simulink model "MagnetoShield_LQ_SIMO_DUE"  (R2019a)
settings: Solver=FixedStepAuto  StartTime=0.0  StopTime=15  RelTol=1e-3  EnableMultiTasking=on
values from neighbouring files (symbols this model uses):
  A = modeld.a    [MagnetoShield_LQ_SIMO_Initialization.m]
  B = modeld.b    [MagnetoShield_LQ_SIMO_Initialization.m]
  C = modeld.c    [MagnetoShield_LQ_SIMO_Initialization.m]
  Ck = [1 0 0;0 0 1]    [MagnetoShield_LQ_SIMO_Initialization.m]
  Dk = [0;0]    [MagnetoShield_LQ_SIMO_Initialization.m]
  K = dlqr(Ai,Bi,Qlq,Rlq)    [MagnetoShield_LQ_SIMO_Initialization.m]
  R = diag([1.5815e-10,6.6217e-09])    [MagnetoShield_LQ_SIMO_Initialization.m]
  Ts = 0.0015    [MagnetoShield_LQ_SIMO_Initialization.m]
undefined symbols (not defined in the file or in its folder): DiscIntNeverNeededParam, Discrete, i0, sigbuilder_block, Time, u0, y0
libraries: MagnetoLibrary x3, ctrlSharedLib x1
settings Model: SimulationMode=external  ExtModeTrigDuration=2  Creator=Jakub  LastModifiedBy=jakub
settings OptimizationCC: EnhancedBackFolding=on  PassReuseOutputArgsAs=Individual arguments  MaxStackSize=64  OptimizeBlockOrder=speed  DifferentSizesBufferReuse=on  OptimizationCustomize=off
settings DebuggingCC: ParameterTunabilityLossMsg=error
settings HardwareCC: ProdBitPerPointer=32  ProdBitPerSizeT=32  ProdBitPerPtrDiffT=32  ProdLargestAtomicInteger=Long  ProdLargestAtomicFloat=Double  ProdWordSize=32  ProdHWDeviceType=ARM Compatible->ARM Cortex
settings SFSimCC: MATLABDynamicMemAlloc=off
settings RTWCC: SystemTargetFile=ert.tlc  HardwareBoard=Arduino Due  TLCOptions=-aInlineSetEventsForThisBaseRateFcn=TLC_FALSE -aSuppressMultiTaskScheduler=TLC_FALSE -aRateBasedStepFcn=1  TemplateMakefile=ert_default_tmf  GenerateReport=on  Toolchain=Arduino ARM  BuildConfiguration=Faster Runs  IncludeHyperlinkInReport=on  LaunchReport=on  GenerateTraceInfo=on  GenerateTraceReport=on  GenerateTraceReportSl=on  GenerateTraceReportSf=on  GenerateTraceReportEml=on
settings CodeAppCC: ForceParamTrailComments=on  IgnoreCustomStorageClasses=off  OperatorAnnotations=on  SimulinkDataObjDesc=on  SFDataObjDesc=on  InsertBlockDesc=on
settings ERTTargetCC: SupportContinuousTime=on  SupportVariableSizeSignals=on  ExtModeStaticAllocSize=24576

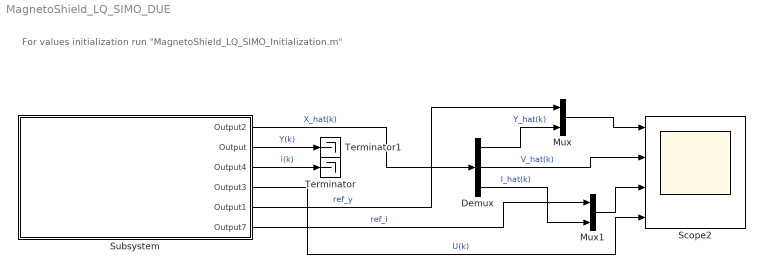
== system MagnetoShield_LQ_SIMO_DUE ==
  note: For values initialization run "MagnetoShield_LQ_SIMO_Initialization.m"
  Demux : Demux  Outputs=3
  Mux : Mux  Inputs=2
  Mux1 : Mux  Inputs=2
  Scope2 : Scope  NumInputPorts=4
  Subsystem : Subsystem
  Terminator : Terminator
  Terminator1 : Terminator
  wires:
  Subsystem/2(Output) -> Terminator1/1  "Y(k)"
  Demux/2 -> Scope2/2  "V_hat(k)"
  Demux/3 -> Mux1/2  "I_hat(k)"
  Mux1/1 -> Scope2/3
  Mux/1 -> Scope2/1
  Demux/1 -> Mux/2  "Y_hat(k)"
  Subsystem/1(Output2) -> Demux/1  "X_hat(k)"
  Subsystem/4(Output3) -> Scope2/4  "U(k)"
  Subsystem/6(Output7) -> Mux1/1  "ref_i"
  Subsystem/5(Output1) -> Mux/1  "ref_y"
  Subsystem/3(Output4) -> Terminator/1  "i(k)"

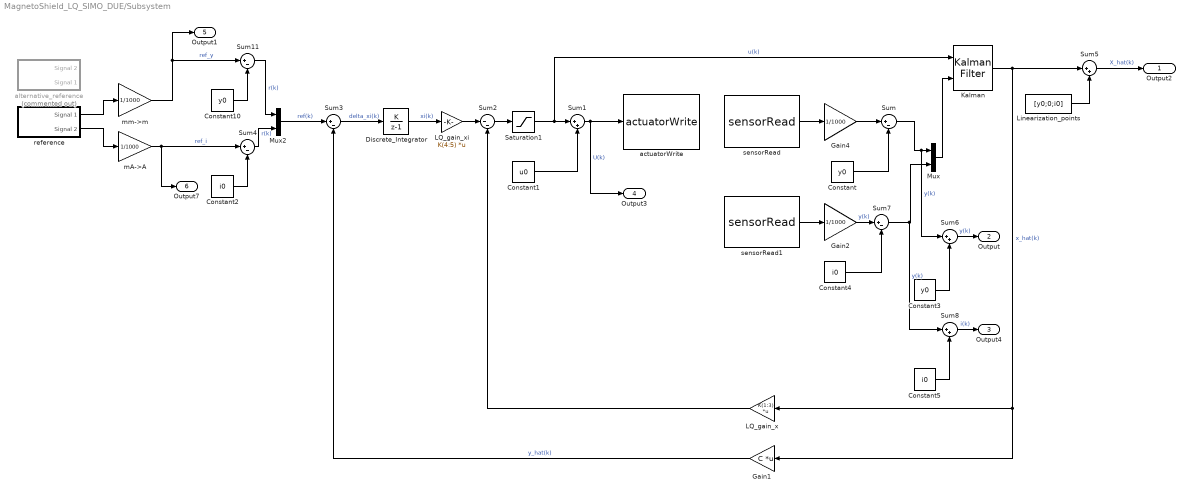
== system MagnetoShield_LQ_SIMO_DUE/Subsystem ==
  Constant : Constant  Value=y0
  Constant1 : Constant  Value=u0
  Constant10 : Constant  Value=y0
  Constant2 : Constant  Value=i0
  Constant3 : Constant  Value=y0
  Constant4 : Constant  Value=i0
  Constant5 : Constant  Value=i0
  Discrete_Integrator : DiscreteIntegrator  IntegratorMethod=Accumulation: Forward Euler  SampleTime=Ts  LimitOutput=on  UpperSaturationLimit=1  LowerSaturationLimit=-1  ICPrevOutput=DiscIntNeverNeededParam  ICPrevScaledInput=DiscIntNeverNeededParam
  Gain1 : Gain  Gain=C  Multiplication=Matrix(K*u)
  Gain2 : Gain  Gain=1/1000
  Gain4 : Gain  Gain=1/1000
  Kalman : ctrlSharedLib/Kalman Filter  TimeDomain=Discrete-Time  UseCurrentEstimator=on  ModelSource=Individual A, B, C, D matrices  ModelSourceVariable=ss(0.95,1,1,0,1)  A=A  B=B  C=Ck  D=Dk  NumberOfStates=1  NumberOfInputs=1  NumberOfOutputs=1  InitialEstimateSource=Dialog  X0=[0.017-y0;0;0-i0]  P0=10  UseK=off  UseGH=off  NumberOfProcessNoiseInputs=1  G=1  TimeInvariantG=on  H=0  TimeInvariantH=on  Q=Q  TimeInvariantQ=on  R=R  TimeInvariantR=on  N=0  TimeInvariantN=on  AddInputPort=on  AddEnablePort=off  OutputEstimatedY=off  OutputP=off  Ts=-1
  LQ_gain_x : Gain  Gain=K(1:3)  Multiplication=Matrix(K*u)
  LQ_gain_xi : Gain  Gain=K(4:5)  Multiplication=Matrix(K*u)
  Linearization_points : Constant  Value=[y0;0;i0]
  Mux : Mux  Inputs=2
  Mux2 : Mux  Inputs=2
  Saturation1 : Saturate  UpperLimit=10-u0  LowerLimit=0-u0
  Sum{,3..4,7,11} (5 alike) : Sum  Inputs=|+-
  Sum{1,5..6,8} (4 alike) : Sum  Inputs=|++
  Sum2 : Sum  Inputs=|--
  actuatorWrite : MagnetoLibrary/actuatorWrite  Board=DUE  Units=Volts
      settings: SourceProductName=AutomationShield
  alternative_reference : Subsystem  Tag=STV Subsys  Commented=on  LoadFcn=sigbuilder_block('load');  StartFcn=sigbuilder_block('start');  StopFcn=sigbuilder_block('stop');  ClipboardFcn=sigbuilder_block('clipboard');  mask(Sigbuilder block){tuvar=[0:10]}
      mask help: Simulink:masks:SigbuilderBlock_MD
      mask init:
      | if ~strcmp(get_param(bdroot(gcbh),'SimulationStatus'),'stopped') tuvar = sigbuilder_block('maskInit'); end
      settings: CopyFcn=sigbuilder_block('copy');  DeleteFcn=sigbuilder_block('delete');  ModelCloseFcn=sigbuilder_block('modelClose');  PreSaveFcn=sigbuilder_block('preSave');  PauseFcn=sigbuilder_block('pause');  ContinueFcn=sigbuilder_block('continue');  NameChangeFcn=sigbuilder_block('namechange');  OpenFcn=sigbuilder_block('open',[434.4 169.8 550.8 400.2 ]);  CloseFcn=sigbuilder_block('close');
      mask Display: plot(0, 0, 100, 100,[2, 2, 32, 32, 2], [68, 8, 8, 68, 68],[32, 2], [38, 38], [32, 19, 2],[53, 60, 44], [32, 17, 17, 2],[16, 16, 31, 31]);txt = getActiveGroup(gcbh);text(2, 100, txt,'verticalAlignment', 'top');
  mA->A : Gain  Gain=1/1000
  mm->m : Gain  Gain=1/1000
  reference : Subsystem  Tag=STV Subsys  LoadFcn=sigbuilder_block('load');  StartFcn=sigbuilder_block('start');  StopFcn=sigbuilder_block('stop');  ClipboardFcn=sigbuilder_block('clipboard');  mask(Sigbuilder block){tuvar=[0:10]}
      mask help: Simulink:masks:SigbuilderBlock_MD
      mask init:
      | if ~strcmp(get_param(bdroot(gcbh),'SimulationStatus'),'stopped') tuvar = sigbuilder_block('maskInit'); end
      settings: CopyFcn=sigbuilder_block('copy');  DeleteFcn=sigbuilder_block('delete');  ModelCloseFcn=sigbuilder_block('modelClose');  PreSaveFcn=sigbuilder_block('preSave');  PauseFcn=sigbuilder_block('pause');  ContinueFcn=sigbuilder_block('continue');  NameChangeFcn=sigbuilder_block('namechange');  OpenFcn=sigbuilder_block('open',[434.4 169.8 550.8 400.2 ]);  CloseFcn=sigbuilder_block('close');
      mask Display: plot(0, 0, 100, 100,[2, 2, 32, 32, 2], [68, 8, 8, 68, 68],[32, 2], [38, 38], [32, 19, 2],[53, 60, 44], [32, 17, 17, 2],[16, 16, 31, 31]);txt = getActiveGroup(gcbh);text(2, 100, txt,'verticalAlignment', 'top');
  sensorRead : MagnetoLibrary/sensorRead  board=DUE  sensor=Distance [mm]  sampling=Ts
      settings: SourceProductName=AutomationShield
  sensorRead1 : MagnetoLibrary/sensorRead  board=DUE  sensor=Current [mA]  sampling=Ts
      settings: SourceProductName=AutomationShield
  Output2 : Outport
  Output : Outport  Port=2
  Output4 : Outport  Port=3
  Output3 : Outport  Port=4
  Output1 : Outport  Port=5
  Output7 : Outport  Port=6
  wires:
  Kalman/1 -> LQ_gain_x/1, Gain1/1, Sum5/1  "x_hat(k)"
  Gain4/1 -> Sum/1
  Sum1/1 -> actuatorWrite/1, Output3/1  "U(k)"
  sensorRead/1 -> Gain4/1
  LQ_gain_xi/1 -> Sum2/1
  Sum2/1 -> Saturation1/1
  LQ_gain_x/1 -> Sum2/2
  Constant/1 -> Sum/2
  Saturation1/1 -> Kalman/1, Sum1/1  "u(k)"
  Sum/1 -> Sum6/1, Mux/1  "y(k)"
  Constant1/1 -> Sum1/2
  Sum3/1 -> Discrete_Integrator/1  "delta_xi(k)"
  Gain1/1 -> Sum3/2  "y_hat(k)"
  Linearization_points/1 -> Sum5/2
  Discrete_Integrator/1 -> LQ_gain_xi/1  "xi(k)"
  Sum5/1 -> Output2/1  "X_hat(k)"
  sensorRead1/1 -> Gain2/1
  Constant4/1 -> Sum7/2
  Sum6/1 -> Output/1  "y(k)"
  Constant3/1 -> Sum6/2
  Mux/1 -> Kalman/2
  Constant5/1 -> Sum8/2
  Sum8/1 -> Output4/1  "i(k)"
  Sum7/1 -> Sum8/1, Mux/2  "y(k)"
  Gain2/1 -> Sum7/1  "y(k)"
  Sum4/1 -> Mux2/2  "r(k)"
  Constant2/1 -> Sum4/2
  Sum11/1 -> Mux2/1  "r(k)"
  Mux2/1 -> Sum3/1  "ref(k)"
  mm->m/1 -> Sum11/1, Output1/1  "ref_y"
  Constant10/1 -> Sum11/2
  mA->A/1 -> Sum4/1, Output7/1  "ref_i"
  reference/2(Signal 2) -> mA->A/1
  reference/1(Signal 1) -> mm->m/1

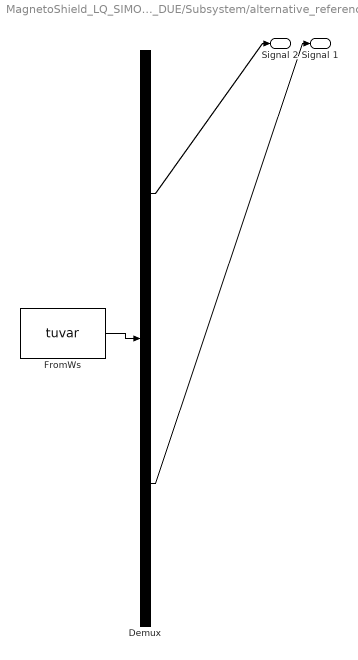
== system MagnetoShield_LQ_SIMO_DUE/Subsystem/alternative_reference ==
  Demux : Demux  Tag=STV Demux  Outputs=2
  FromWs : FromWorkspace  Tag=STV FromWs  VariableName=tuvar  SampleTime=0
      SigBuilderData=|
      | common.afterFinalStr = 'Extrapolate'
      | common.sampleTime = 0
      | dataSet.timeRange = [0 15]
      | dataSet.name = 'Group 1'
      | sbobj.Groups.Name = 'Group 1'
      | sbobj.Groups.Signals(1).Name = 'Signal 2'
      | sbobj.Groups.Signals(1).XData = [0 7.5 7.5 15]
      | sbobj.Groups.Signals(1).YData = [14 14 16 16]
      | sbobj.Groups.Signals(2).Name = 'Signal 1'
      | sbobj.Groups.Signals(2).XData = [0 7.5 7.5 15]
      | sbobj.Groups.Signals(2).YData = [20 20 35 35]
      | sbobj.Groups.TimeRange = [0 15]
  Signal 2 : Outport  Tag=STV Outport
  Signal 1 : Outport  Tag=STV Outport  Port=2
  wires:
  FromWs/1 -> Demux/1
  Demux/1 -> Signal 2/1
  Demux/2 -> Signal 1/1

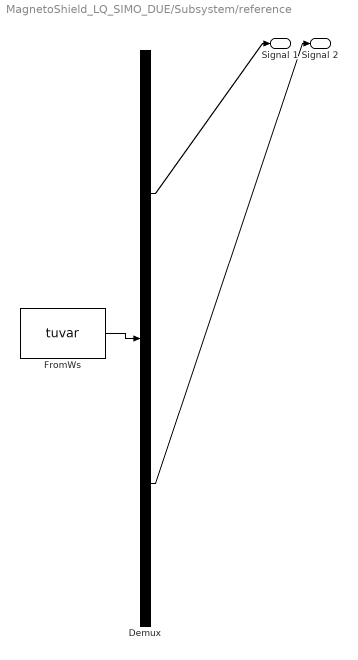
== system MagnetoShield_LQ_SIMO_DUE/Subsystem/reference ==
  Demux : Demux  Tag=STV Demux  Outputs=2
  FromWs : FromWorkspace  Tag=STV FromWs  VariableName=tuvar  SampleTime=0
      SigBuilderData=|
      | common.afterFinalStr = 'Extrapolate'
      | common.sampleTime = 0
      | dataSet.timeRange = [0 15]
      | dataSet.name = 'Group 1'
      | sbobj.Groups.Name = 'Group 1'
      | sbobj.Groups.Signals(1).Name = 'Signal 1'
      | sbobj.Groups.Signals(1).XData = [0 2 4 6 8 10 12 14 15]
      | sbobj.Groups.Signals(1).YData = [14 14 15 14.5 14.5 14.5 14.5 14.5 14.5]
      | sbobj.Groups.Signals(2).Name = 'Signal 2'
      | sbobj.Groups.Signals(2).XData = [0 2 4 6 8 10 12 14 15]
      | sbobj.Groups.Signals(2).YData = [18 18 18 18 18 25 21 21 21]
      | sbobj.Groups.TimeRange = [0 15]
  Signal 1 : Outport  Tag=STV Outport
  Signal 2 : Outport  Tag=STV Outport  Port=2
  wires:
  Demux/2 -> Signal 2/1
  Demux/1 -> Signal 1/1
  FromWs/1 -> Demux/1
